simulink model "Problem8"  (R2020a)
settings: Solver=VariableStepAuto  StartTime=0.0  StopTime=10.0  RelTol=1e-3
settings Model: Creator=sreeram  LastModifiedBy=sreeram

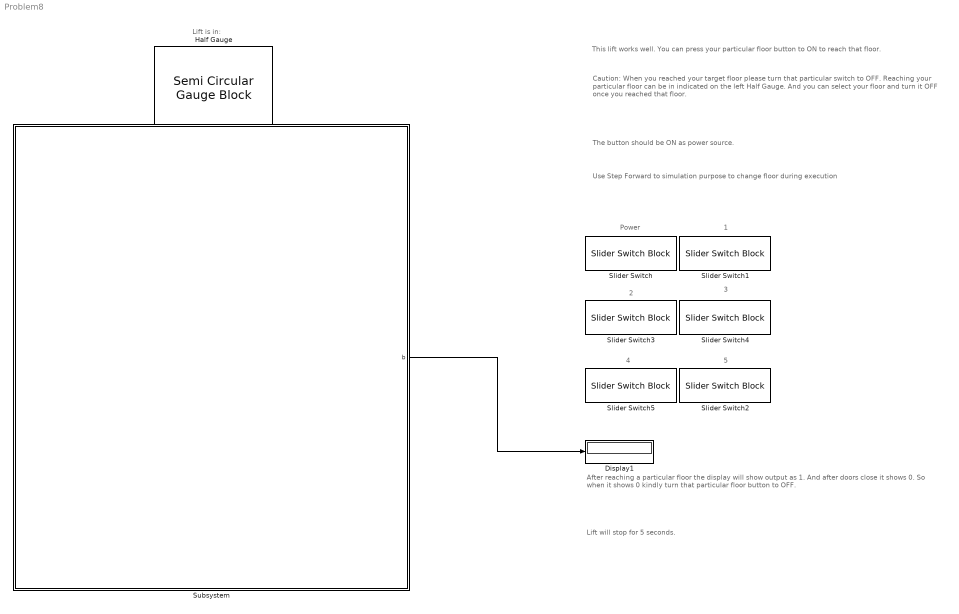
== system Problem8 ==
  note: Lift will stop for 5 seconds.
  note: After reaching a particular floor the display will show output as 1.
      | And after doors close it shows 0. So when it shows 0 kindly turn that particular floor button to OFF.
  note: Use Step Forward to simulation purpose to change floor during execution
  note: Lift is in:
  note: 5
  note: 4
  note: 3
  note: 2
  note: 1
  note: Power
  note: Caution: When you reached your target floor please turn that particular switch to OFF.
      | Reaching your particular floor can be in indicated on the left Half Gauge.
      | And you can select your floor and turn it OFF once you reached that floor.
  note: The button should be ON as power source.
  note: This lift works well. You can press your particular floor button to ON to reach that floor.
  Display1 : Display
  Half Gauge : SemiCircularGaugeBlock  LabelPosition=Bottom  ScaleMax=5  TickInterval=1
  Slider Switch{,1..5} (6 alike) : SliderSwitchBlock
      settings: Values={{'Off', 'On'}, [0 1]}
  Subsystem : Subsystem
      mask Display: image('C:\Users\sreeram\Desktop\automatic-elevator-door-500x500.jpg'); % Use "Edit Image" on toolstrip to change.
  wires:
  Subsystem/1(b) -> Display1/1

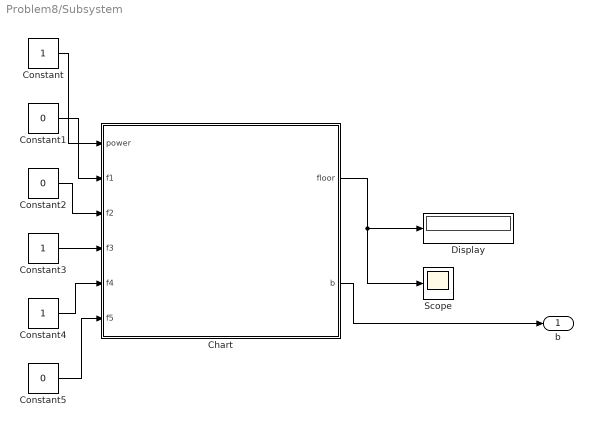
== system Problem8/Subsystem ==
  Chart : Stateflow chart  TreatAsAtomicUnit=on
  Constant : Constant
  Constant1 : Constant  Value=0
  Constant2 : Constant  Value=0
  Constant3 : Constant
  Constant4 : Constant
  Constant5 : Constant  Value=0
  Display : Display
  Scope : Scope
  b : Outport
  wires:
  Chart/2(b) -> b/1
  Constant3/1 -> Chart/4(f3)
  Constant4/1 -> Chart/5(f4)
  Constant2/1 -> Chart/3(f2)
  Chart/1(floor) -> Scope/1, Display/1
  Constant5/1 -> Chart/6(f5)
  Constant/1 -> Chart/1(power)
  Constant1/1 -> Chart/2(f1)

== stateflow chart Problem8/Subsystem/Chart ==
  state lift_off
  state lift_on
    du: t = t + 1;
    (history)
    state floor
      en:f1, f2, f3, f4, f5;
      t = 0;
      b = 0;
    state floor1
      en: t = 0;
      floor = 1;n = 5;
      b = 1;
    state floor2
      en: t = 0;
      floor = 2; n = 5;
      b = 1;
    state floor3
      en: t = 0;
      floor = 3; n = 5;
      b = 1;
    state floor4
      en: t = 0;
      floor = 4;n = 5;
      b = 1;
    state floor5
      en: t = 0;
      floor = 5;n=5;
      b = 1;
    floor5 -> floor : [t == n]
    floor4 -> floor : [t == n]
    floor -> floor4 [order 4] : [f4 == 1]
    floor -> floor2 [order 2] : [f2 == 1]
    (default) -> floor
    floor2 -> floor : [t == n]
    floor -> floor1 [order 1] : [f1 == 1]
    floor1 -> floor : [t == n]
    floor -> floor3 [order 3] : [f3 ==1]
    floor3 -> floor : [t == n]
    floor -> floor5 [order 5] : [f5 == 1]
  (default) -> lift_off
  lift_off -> lift_on : [power == 1]
  lift_on -> lift_off : [power == 0]
  data: power input; f1 input; f2 input; f3 input; f4 input; f5 input; t local; floor output; n local; b output
